simulink model "commands_to_xplane10_R2011b"  (Simulink 8.4)
settings: Solver=FixedStepDiscrete  StartTime=0.0  StopTime=inf  FixedStep=1/100  RelTol=1e-3
libraries: etargetslib x1, dspnetwork x1
settings Model: Creator=Mohamed Abdelkader  LastModifiedBy=abdkadma
settings DataIOCC: SignalLoggingSaveFormat=Dataset
settings OptimizationCC: SimCompilerOptimization=On
settings DebuggingCC: FcnCallInpInsideContextMsg=EnableAllAsWarning
settings ConfigurationSet: Description=SimMechanics 2G

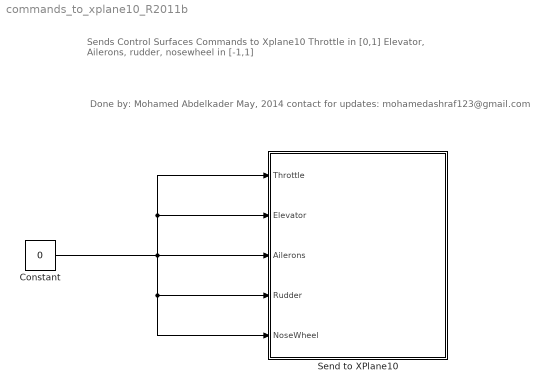
== system commands_to_xplane10_R2011b ==
  note: Done by: Mohamed Abdelkader
      | May, 2014
      | contact for updates: mohamedashraf123@gmail.com
  note: Sends Control Surfaces Commands to Xplane10
      | Throttle in [0,1]
      | Elevator, Ailerons, rudder, nosewheel in [-1,1]
  Constant : Constant  Value=0  OutDataTypeStr=single
  Send to XPlane10 : Subsystem  Description=|  mask(Send Commands to X-Plane 10){remoteURL='127.0.0.1', remotePort=49000}
      | Done by: Mohamed Abdelkader
      | Contact for updates: mohamedashraf123@gmail.com
      mask prompts: remoteURL "Remote IP address (default='127.0.0.1'): X-Plane10 IP"; remotePort "Remote IP port:X-Plane10 port(default=49000)"
      mask help:
      | Sends Control Surfaces Commands to Xplane10
      | Throttle in [0,1]
      | Elevator, Ailerons, rudder, nosewheel in [-1,1]
      mask TypeOptions remoteURL: UDP Send/remoteURL
      mask TypeOptions remotePort: UDP Send/remotePort
  wires:
  Constant/1 -> Send to XPlane10/3(Ailerons), Send to XPlane10/5(NoseWheel), Send to XPlane10/4(Rudder), Send to XPlane10/2(Elevator), Send to XPlane10/1(Throttle)

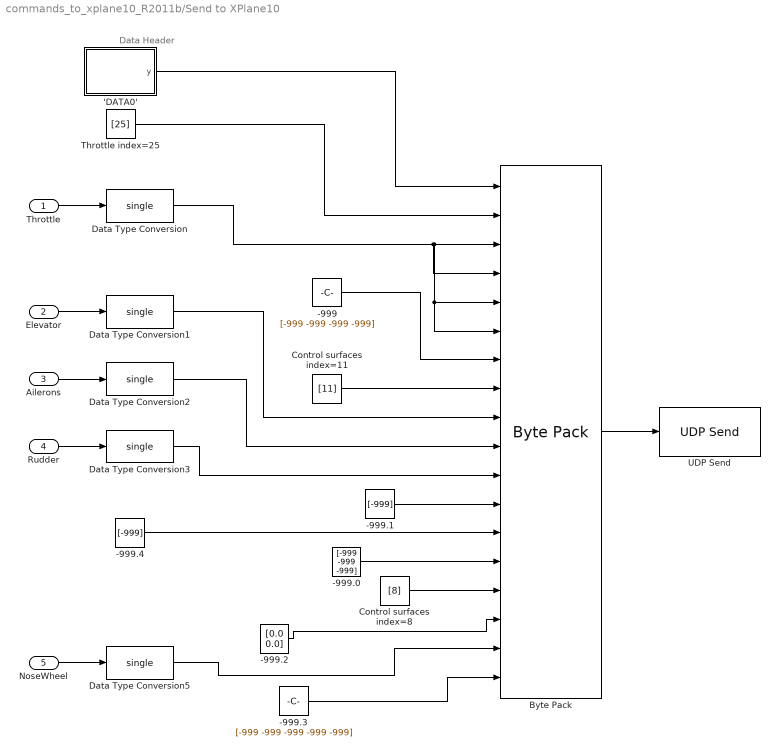
== system commands_to_xplane10_R2011b/Send to XPlane10 ==
  note: Data Header
  Throttle : Inport
  Elevator : Inport  Port=2
  Ailerons : Inport  Port=3
  Rudder : Inport  Port=4
  NoseWheel : Inport  Port=5
  'DATA0' : MATLAB Function  TreatAsAtomicUnit=on
  -999 : Constant  Value=[-999 -999 -999 -999]  OutDataTypeStr=int32  SampleTime=-1
  -999.0 : Constant  Value=[-999 -999 -999]  OutDataTypeStr=int32  SampleTime=-1
  -999.1 : Constant  Value=[-999]  OutDataTypeStr=int32  SampleTime=-1
  -999.2 : Constant  Value=[0.0 0.0]  OutDataTypeStr=single  SampleTime=-1
  -999.3 : Constant  Value=[-999 -999 -999 -999 -999]  OutDataTypeStr=int32  SampleTime=-1
  -999.4 : Constant  Value=[-999]  OutDataTypeStr=single  SampleTime=-1
  Byte Pack : etargetslib/Byte Pack  datatypes={'uint8','uint32','single','single','single','single','int32','uint32','single','single','single','int32','single','int32','uint32','single','single','int32'}  byteAlign=1
  Control surfaces index=11 : Constant  Value=[11]  OutDataTypeStr=uint32  SampleTime=-1
  Control surfaces index=8 : Constant  Value=[8]  OutDataTypeStr=uint32  SampleTime=-1
  Data Type Conversion : DataTypeConversion  OutMin=[0]  OutMax=[1.0]  OutDataTypeStr=single
  Data Type Conversion{1..3,5} (4 alike) : DataTypeConversion  OutMin=[-1.0]  OutMax=[1.0]  OutDataTypeStr=single
  Throttle index=25 : Constant  Value=[25]  OutDataTypeStr=uint32  SampleTime=-1
  UDP Send : dspnetwork/UDP Send  remoteURL=remoteURL  remotePort=remotePort  localURL='0.0.0.0'  localPortSource=Automatically determine  localPort=-1  sampletime=-1  separateLengthPort=0
  wires:
  Ailerons/1 -> Data Type Conversion2/1
  Control surfaces index=11/1 -> Byte Pack/8
  Throttle/1 -> Data Type Conversion/1
  Data Type Conversion1/1 -> Byte Pack/9
  'DATA0'/1(y) -> Byte Pack/1
  Throttle index=25/1 -> Byte Pack/2
  Byte Pack/1 -> UDP Send/1
  -999/1 -> Byte Pack/7
  Data Type Conversion2/1 -> Byte Pack/10
  Data Type Conversion3/1 -> Byte Pack/11
  Rudder/1 -> Data Type Conversion3/1
  -999.0/1 -> Byte Pack/14
  Elevator/1 -> Data Type Conversion1/1
  Data Type Conversion/1 -> Byte Pack/3, Byte Pack/6, Byte Pack/5, Byte Pack/4
  -999.1/1 -> Byte Pack/12
  Control surfaces index=8/1 -> Byte Pack/15
  -999.2/1 -> Byte Pack/16
  Data Type Conversion5/1 -> Byte Pack/17
  NoseWheel/1 -> Data Type Conversion5/1
  -999.3/1 -> Byte Pack/18
  -999.4/1 -> Byte Pack/13

== matlab function Send to XPlane10/'DATA0' ==
  data: y output double
function y = fcn()
%#codegen
%y=uint8(zeros(1,77));
y = uint8('DATA0');
